simulink library "CAN_EV_lib"  (Simulink 7.5)
settings: Solver=ode45  StartTime=0.0  StopTime=10.0  RelTol=1e-3
values from neighbouring files (symbols this model uses):
  pOUTP_st_ChrgrPlugSwtACChrg_C = Simulink.Parameter    [CAN_par.m]
  pOUTP_st_ChrgrPlugSwtDCChrg_C = Simulink.Parameter    [CAN_par.m]
  pOUTP_st_ChrgrPlugSwtNoChrg_C = Simulink.Parameter    [CAN_par.m]
libraries: BaseOperationLib_Browser x6, simulink x1
settings Model: Creator=wuaibin  LastModifiedBy=wuaibin

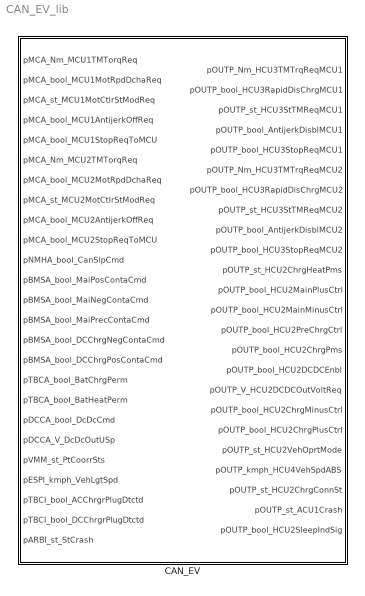
== system CAN_EV_lib ==
  CAN_EV : Subsystem

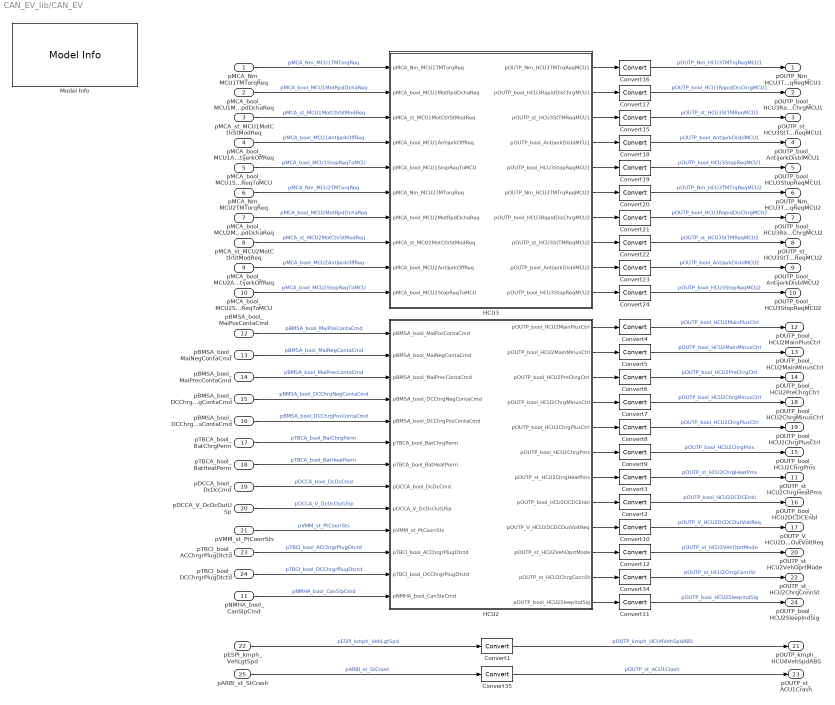
== system CAN_EV_lib/CAN_EV ==
  pMCA_Nm_MCU1TMTorqReq : Inport  OutDataType=fixdt(1, 16)  OutScaling=2^0
  pMCA_bool_MCU1MotRpdDchaReq : Inport  Port=2  OutDataType=fixdt(1, 16)  OutScaling=2^0
  pMCA_st_MCU1MotCtlrStModReq : Inport  Port=3  OutDataType=fixdt(1, 16)  OutScaling=2^0
  pMCA_bool_MCU1AntijerkOffReq : Inport  Port=4  OutDataType=fixdt(1, 16)  OutScaling=2^0
  pMCA_bool_MCU1StopReqToMCU : Inport  Port=5  OutDataType=fixdt(1, 16)  OutScaling=2^0
  pMCA_Nm_MCU2TMTorqReq : Inport  Port=6  OutDataType=fixdt(1, 16)  OutScaling=2^0
  pMCA_bool_MCU2MotRpdDchaReq : Inport  Port=7  OutDataType=fixdt(1, 16)  OutScaling=2^0
  pMCA_st_MCU2MotCtlrStModReq : Inport  Port=8  OutDataType=fixdt(1, 16)  OutScaling=2^0
  pMCA_bool_MCU2AntijerkOffReq : Inport  Port=9  OutDataType=fixdt(1, 16)  OutScaling=2^0
  pMCA_bool_MCU2StopReqToMCU : Inport  Port=10  OutDataType=fixdt(1, 16)  OutScaling=2^0
  pNMHA_bool_CanSlpCmd : Inport  Port=11  OutDataType=fixdt(1, 16)  OutScaling=2^0
  pBMSA_bool_MaiPosContaCmd : Inport  Port=12  OutDataType=fixdt(1, 16)  OutScaling=2^0
  pBMSA_bool_MaiNegContaCmd : Inport  Port=13  OutDataType=fixdt(1, 16)  OutScaling=2^0
  pBMSA_bool_MaiPrecContaCmd : Inport  Port=14  OutDataType=fixdt(1, 16)  OutScaling=2^0
  pBMSA_bool_DCChrgNegContaCmd : Inport  Port=15  OutDataType=fixdt(1, 16)  OutScaling=2^0
  pBMSA_bool_DCChrgPosContaCmd : Inport  Port=16  OutDataType=fixdt(1, 16)  OutScaling=2^0
  pTBCA_bool_BatChrgPerm : Inport  Port=17  OutDataType=fixdt(1, 16)  OutScaling=2^0
  pTBCA_bool_BatHeatPerm : Inport  Port=18  OutDataType=fixdt(1, 16)  OutScaling=2^0
  pDCCA_bool_DcDcCmd : Inport  Port=19  OutDataType=fixdt(1, 16)  OutScaling=2^0
  pDCCA_V_DcDcOutUSp : Inport  Port=20  OutDataType=fixdt(1, 16)  OutScaling=2^0
  pVMM_st_PtCoorrSts : Inport  Port=21  OutDataType=fixdt(1, 16)  OutScaling=2^0
  pESPI_kmph_VehLgtSpd : Inport  Port=22
  pTBCI_bool_ACChrgrPlugDtctd : Inport  Port=23  OutDataType=fixdt(1, 16)  OutScaling=2^0
  pTBCI_bool_DCChrgrPlugDtctd : Inport  Port=24  OutDataType=fixdt(1, 16)  OutScaling=2^0
  pARBI_st_StCrash : Inport  Port=25
  Convert{1..12,15..24,34..35} (24 alike) : DataTypeConversion  OutDataType=fixdt(1, 16)  OutScaling=2^0
  HCU2 : Subsystem
  HCU3 : Subsystem
  Model Info : simulink/Model-Wide Utilities/Model Info  SystemSampleTime=-1  InitialBlockCM=None  BlockCM=None  Frame=on  DisplayStringWithTags=Model Info\nCreated: %<Created>\nCreator: wuaibin  HorizontalTextAlignment=Center  LeftAlignmentValue=0.5  SourceBlockDiagram=HQEV_HCU  TagMaxNumber=20
  pOUTP_Nm_HCU3TMTrqReqMCU1 : Outport
  pOUTP_bool_HCU3RapidDisChrgMCU1 : Outport  Port=2
  pOUTP_st_HCU3StTMReqMCU1 : Outport  Port=3
  pOUTP_bool_AntijerkDisblMCU1 : Outport  Port=4
  pOUTP_bool_HCU3StopReqMCU1 : Outport  Port=5
  pOUTP_Nm_HCU3TMTrqReqMCU2 : Outport  Port=6
  pOUTP_bool_HCU3RapidDisChrgMCU2 : Outport  Port=7
  pOUTP_st_HCU3StTMReqMCU2 : Outport  Port=8
  pOUTP_bool_AntijerkDisblMCU2 : Outport  Port=9
  pOUTP_bool_HCU3StopReqMCU2 : Outport  Port=10
  pOUTP_st_HCU2ChrgHeatPms : Outport  Port=11  OutDataType=fixdt(1, 16)  OutScaling=2^0
  pOUTP_bool_HCU2MainPlusCtrl : Outport  Port=12  OutDataType=fixdt(1, 16)  OutScaling=2^0
  pOUTP_bool_HCU2MainMinusCtrl : Outport  Port=13  OutDataType=fixdt(1, 16)  OutScaling=2^0
  pOUTP_bool_HCU2PreChrgCtrl : Outport  Port=14  OutDataType=fixdt(1, 16)  OutScaling=2^0
  pOUTP_bool_HCU2ChrgPms : Outport  Port=15  OutDataType=fixdt(1, 16)  OutScaling=2^0
  pOUTP_bool_HCU2DCDCEnbl : Outport  Port=16  OutDataType=fixdt(1, 16)  OutScaling=2^0
  pOUTP_V_HCU2DCDCOutVoltReq : Outport  Port=17  OutDataType=fixdt(1, 16)  OutScaling=2^0
  pOUTP_bool_HCU2ChrgMinusCtrl : Outport  Port=18  OutDataType=fixdt(1, 16)  OutScaling=2^0
  pOUTP_bool_HCU2ChrgPlusCtrl : Outport  Port=19  OutDataType=fixdt(1, 16)  OutScaling=2^0
  pOUTP_st_HCU2VehOprtMode : Outport  Port=20  OutDataType=fixdt(1, 16)  OutScaling=2^0
  pOUTP_kmph_HCU4VehSpdABS : Outport  Port=21
  pOUTP_st_HCU2ChrgConnSt : Outport  Port=22  OutDataType=fixdt(1, 16)  OutScaling=2^0
  pOUTP_st_ACU1Crash : Outport  Port=23
  pOUTP_bool_HCU2SleepIndSig : Outport  Port=24  OutDataType=fixdt(1, 16)  OutScaling=2^0
  wires:
  Convert11/1 -> pOUTP_bool_HCU2SleepIndSig/1  "pOUTP_bool_HCU2SleepIndSig"
  HCU2/12(pOUTP_bool_HCU2SleepIndSig) -> Convert11/1
  pNMHA_bool_CanSlpCmd/1 -> HCU2/13(pNMHA_bool_CanSlpCmd)  "pNMHA_bool_CanSlpCmd"
  pARBI_st_StCrash/1 -> Convert35/1  "pARBI_st_StCrash"
  Convert35/1 -> pOUTP_st_ACU1Crash/1  "pOUTP_st_ACU1Crash"
  Convert24/1 -> pOUTP_bool_HCU3StopReqMCU2/1  "pOUTP_bool_HCU3StopReqMCU2"
  Convert23/1 -> pOUTP_bool_AntijerkDisblMCU2/1  "pOUTP_bool_AntijerkDisblMCU2"
  Convert22/1 -> pOUTP_st_HCU3StTMReqMCU2/1  "pOUTP_st_HCU3StTMReqMCU2"
  Convert21/1 -> pOUTP_bool_HCU3RapidDisChrgMCU2/1  "pOUTP_bool_HCU3RapidDisChrgMCU2"
  Convert20/1 -> pOUTP_Nm_HCU3TMTrqReqMCU2/1  "pOUTP_Nm_HCU3TMTrqReqMCU2"
  Convert19/1 -> pOUTP_bool_HCU3StopReqMCU1/1  "pOUTP_bool_HCU3StopReqMCU1"
  Convert18/1 -> pOUTP_bool_AntijerkDisblMCU1/1  "pOUTP_bool_AntijerkDisblMCU1"
  Convert15/1 -> pOUTP_st_HCU3StTMReqMCU1/1  "pOUTP_st_HCU3StTMReqMCU1"
  Convert17/1 -> pOUTP_bool_HCU3RapidDisChrgMCU1/1  "pOUTP_bool_HCU3RapidDisChrgMCU1"
  Convert16/1 -> pOUTP_Nm_HCU3TMTrqReqMCU1/1  "pOUTP_Nm_HCU3TMTrqReqMCU1"
  Convert12/1 -> pOUTP_st_HCU2VehOprtMode/1  "pOUTP_st_HCU2VehOprtMode"
  Convert10/1 -> pOUTP_V_HCU2DCDCOutVoltReq/1  "pOUTP_V_HCU2DCDCOutVoltReq"
  Convert9/1 -> pOUTP_bool_HCU2ChrgPms/1  "pOUTP_bool_HCU2ChrgPms"
  Convert8/1 -> pOUTP_bool_HCU2ChrgPlusCtrl/1  "pOUTP_bool_HCU2ChrgPlusCtrl"
  Convert7/1 -> pOUTP_bool_HCU2ChrgMinusCtrl/1  "pOUTP_bool_HCU2ChrgMinusCtrl"
  Convert6/1 -> pOUTP_bool_HCU2PreChrgCtrl/1  "pOUTP_bool_HCU2PreChrgCtrl"
  Convert5/1 -> pOUTP_bool_HCU2MainMinusCtrl/1  "pOUTP_bool_HCU2MainMinusCtrl"
  Convert4/1 -> pOUTP_bool_HCU2MainPlusCtrl/1  "pOUTP_bool_HCU2MainPlusCtrl"
  Convert3/1 -> pOUTP_st_HCU2ChrgHeatPms/1  "pOUTP_st_HCU2ChrgHeatPms"
  Convert2/1 -> pOUTP_bool_HCU2DCDCEnbl/1  "pOUTP_bool_HCU2DCDCEnbl"
  pTBCI_bool_DCChrgrPlugDtctd/1 -> HCU2/12(pTBCI_bool_DCChrgrPlugDtctd)  "pTBCI_bool_DCChrgrPlugDtctd"
  pTBCI_bool_ACChrgrPlugDtctd/1 -> HCU2/11(pTBCI_bool_ACChrgrPlugDtctd)  "pTBCI_bool_ACChrgrPlugDtctd"
  Convert34/1 -> pOUTP_st_HCU2ChrgConnSt/1  "pOUTP_st_HCU2ChrgConnSt"
  HCU2/11(pOUTP_st_HCU2ChrgConnSt) -> Convert34/1
  Convert1/1 -> pOUTP_kmph_HCU4VehSpdABS/1  "pOUTP_kmph_HCU4VehSpdABS"
  pESPI_kmph_VehLgtSpd/1 -> Convert1/1  "pESPI_kmph_VehLgtSpd"
  HCU2/10(pOUTP_st_HCU2VehOprtMode) -> Convert12/1
  pVMM_st_PtCoorrSts/1 -> HCU2/10(pVMM_st_PtCoorrSts)  "pVMM_st_PtCoorrSts"
  HCU3/7(pOUTP_bool_HCU3RapidDisChrgMCU2) -> Convert21/1
  HCU3/8(pOUTP_st_HCU3StTMReqMCU2) -> Convert22/1
  HCU3/9(pOUTP_bool_AntijerkDisblMCU2) -> Convert23/1
  HCU3/10(pOUTP_bool_HCU3StopReqMCU2) -> Convert24/1
  HCU3/1(pOUTP_Nm_HCU3TMTrqReqMCU1) -> Convert16/1
  HCU3/2(pOUTP_bool_HCU3RapidDisChrgMCU1) -> Convert17/1
  HCU3/3(pOUTP_st_HCU3StTMReqMCU1) -> Convert15/1
  HCU3/4(pOUTP_bool_AntijerkDisblMCU1) -> Convert18/1
  HCU3/5(pOUTP_bool_HCU3StopReqMCU1) -> Convert19/1
  HCU3/6(pOUTP_Nm_HCU3TMTrqReqMCU2) -> Convert20/1
  pMCA_bool_MCU2StopReqToMCU/1 -> HCU3/10(pMCA_bool_MCU2StopReqToMCU)  "pMCA_bool_MCU2StopReqToMCU"
  pMCA_bool_MCU2AntijerkOffReq/1 -> HCU3/9(pMCA_bool_MCU2AntijerkOffReq)  "pMCA_bool_MCU2AntijerkOffReq"
  pMCA_st_MCU2MotCtlrStModReq/1 -> HCU3/8(pMCA_st_MCU2MotCtlrStModReq)  "pMCA_st_MCU2MotCtlrStModReq"
  pMCA_bool_MCU2MotRpdDchaReq/1 -> HCU3/7(pMCA_bool_MCU2MotRpdDchaReq)  "pMCA_bool_MCU2MotRpdDchaReq"
  pMCA_Nm_MCU1TMTorqReq/1 -> HCU3/1(pMCA_Nm_MCU1TMTorqReq)  "pMCA_Nm_MCU1TMTorqReq"
  pMCA_bool_MCU1MotRpdDchaReq/1 -> HCU3/2(pMCA_bool_MCU1MotRpdDchaReq)  "pMCA_bool_MCU1MotRpdDchaReq"
  pMCA_st_MCU1MotCtlrStModReq/1 -> HCU3/3(pMCA_st_MCU1MotCtlrStModReq)  "pMCA_st_MCU1MotCtlrStModReq"
  pMCA_bool_MCU1AntijerkOffReq/1 -> HCU3/4(pMCA_bool_MCU1AntijerkOffReq)  "pMCA_bool_MCU1AntijerkOffReq"
  pMCA_bool_MCU1StopReqToMCU/1 -> HCU3/5(pMCA_bool_MCU1StopReqToMCU)  "pMCA_bool_MCU1StopReqToMCU"
  pMCA_Nm_MCU2TMTorqReq/1 -> HCU3/6(pMCA_Nm_MCU2TMTorqReq)  "pMCA_Nm_MCU2TMTorqReq"
  pBMSA_bool_MaiPosContaCmd/1 -> HCU2/1(pBMSA_bool_MaiPosContaCmd)  "pBMSA_bool_MaiPosContaCmd"
  pBMSA_bool_MaiNegContaCmd/1 -> HCU2/2(pBMSA_bool_MaiNegContaCmd)  "pBMSA_bool_MaiNegContaCmd"
  pBMSA_bool_MaiPrecContaCmd/1 -> HCU2/3(pBMSA_bool_MaiPrecContaCmd)  "pBMSA_bool_MaiPrecContaCmd"
  pTBCA_bool_BatChrgPerm/1 -> HCU2/6(pTBCA_bool_BatChrgPerm)  "pTBCA_bool_BatChrgPerm"
  pTBCA_bool_BatHeatPerm/1 -> HCU2/7(pTBCA_bool_BatHeatPerm)  "pTBCA_bool_BatHeatPerm"
  HCU2/7(pOUTP_st_HCU2ChrgHeatPms) -> Convert3/1
  HCU2/1(pOUTP_bool_HCU2MainPlusCtrl) -> Convert4/1
  HCU2/2(pOUTP_bool_HCU2MainMinusCtrl) -> Convert5/1
  HCU2/3(pOUTP_bool_HCU2PreChrgCtrl) -> Convert6/1
  HCU2/6(pOUTP_bool_HCU2ChrgPms) -> Convert9/1
  HCU2/8(pOUTP_bool_HCU2DCDCEnbl) -> Convert2/1
  HCU2/9(pOUTP_V_HCU2DCDCOutVoltReq) -> Convert10/1
  pDCCA_bool_DcDcCmd/1 -> HCU2/8(pDCCA_bool_DcDcCmd)  "pDCCA_bool_DcDcCmd"
  pDCCA_V_DcDcOutUSp/1 -> HCU2/9(pDCCA_V_DcDcOutUSp)  "pDCCA_V_DcDcOutUSp"
  pBMSA_bool_DCChrgNegContaCmd/1 -> HCU2/4(pBMSA_bool_DCChrgNegContaCmd)  "pBMSA_bool_DCChrgNegContaCmd"
  pBMSA_bool_DCChrgPosContaCmd/1 -> HCU2/5(pBMSA_bool_DCChrgPosContaCmd)  "pBMSA_bool_DCChrgPosContaCmd"
  HCU2/4(pOUTP_bool_HCU2ChrgMinusCtrl) -> Convert7/1
  HCU2/5(pOUTP_bool_HCU2ChrgPlusCtrl) -> Convert8/1

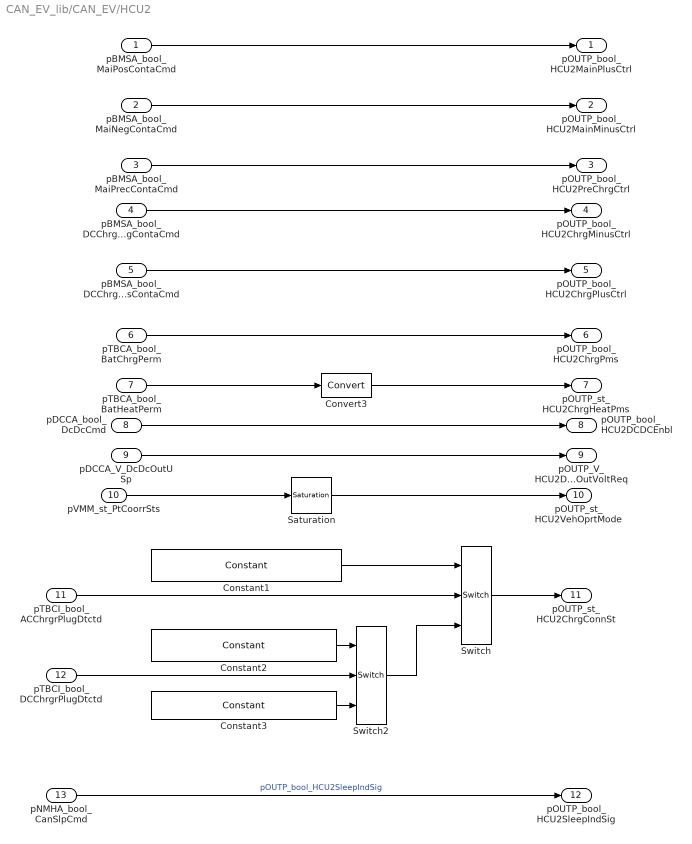
== system CAN_EV_lib/CAN_EV/HCU2 ==
  pBMSA_bool_MaiPosContaCmd : Inport  OutDataType=fixdt(1, 16)  OutScaling=2^0
  pBMSA_bool_MaiNegContaCmd : Inport  Port=2  OutDataType=fixdt(1, 16)  OutScaling=2^0
  pBMSA_bool_MaiPrecContaCmd : Inport  Port=3  OutDataType=fixdt(1, 16)  OutScaling=2^0
  pBMSA_bool_DCChrgNegContaCmd : Inport  Port=4  OutDataType=fixdt(1, 16)  OutScaling=2^0
  pBMSA_bool_DCChrgPosContaCmd : Inport  Port=5  OutDataType=fixdt(1, 16)  OutScaling=2^0
  pTBCA_bool_BatChrgPerm : Inport  Port=6  OutDataType=fixdt(1, 16)  OutScaling=2^0
  pTBCA_bool_BatHeatPerm : Inport  Port=7  OutDataType=fixdt(1, 16)  OutScaling=2^0
  pDCCA_bool_DcDcCmd : Inport  Port=8  OutDataType=fixdt(1, 16)  OutScaling=2^0
  pDCCA_V_DcDcOutUSp : Inport  Port=9  OutDataType=fixdt(1, 16)  OutScaling=2^0
  pVMM_st_PtCoorrSts : Inport  Port=10
  pTBCI_bool_ACChrgrPlugDtctd : Inport  Port=11  OutDataType=fixdt(1, 16)  OutScaling=2^0
  pTBCI_bool_DCChrgrPlugDtctd : Inport  Port=12  OutDataType=fixdt(1, 16)  OutScaling=2^0
  pNMHA_bool_CanSlpCmd : Inport  Port=13  OutDataType=fixdt(1, 16)  OutScaling=2^0
  Constant1 : BaseOperationLib_Browser/Sources&Sinks/Constant  Value=pOUTP_st_ChrgrPlugSwtACChrg_C  OutMin=[]  OutMax=[]  OutDataType=fixdt(1, 16)  ConRadixGroup=Use specified scaling  OutScaling=2^0  OutDataTypeStr=Inherit: Inherit from 'Constant value'
  Constant2 : BaseOperationLib_Browser/Sources&Sinks/Constant  Value=pOUTP_st_ChrgrPlugSwtDCChrg_C  OutMin=[]  OutMax=[]  OutDataType=fixdt(1, 16)  ConRadixGroup=Use specified scaling  OutScaling=2^0  OutDataTypeStr=Inherit: Inherit from 'Constant value'
  Constant3 : BaseOperationLib_Browser/Sources&Sinks/Constant  Value=pOUTP_st_ChrgrPlugSwtNoChrg_C  OutMin=[]  OutMax=[]  OutDataType=fixdt(1, 16)  ConRadixGroup=Use specified scaling  OutScaling=2^0  OutDataTypeStr=Inherit: Inherit from 'Constant value'
  Convert3 : DataTypeConversion  OutDataType=fixdt(1, 16)  OutScaling=2^0
  Saturation : BaseOperationLib_Browser/Discontinuities Unchanged/Saturation  UpperLimit=15  LowerLimit=0  OutMin=[]  OutMax=[]  OutDataType=fixdt(1, 16)  OutScaling=2^0
      settings: AttributesFormatString=ULim:%<UpperLimit>\nLLim:%<LowerLimit>
  Switch : BaseOperationLib_Browser/Signal Routing Changed/Switch  Criteria=u2 ~= 0  Threshold=1  InputSameDT=on  OutMin=[]  OutMax=[]  OutDataType=fixdt(1,16,0)  OutScaling=[]  SaturateOnIntegerOverflow=on
  Switch2 : BaseOperationLib_Browser/Signal Routing Changed/Switch  Criteria=u2 ~= 0  Threshold=1  InputSameDT=on  OutMin=[]  OutMax=[]  OutDataType=fixdt(1,16,0)  OutScaling=[]  SaturateOnIntegerOverflow=on
  pOUTP_bool_HCU2MainPlusCtrl : Outport  OutDataType=fixdt(1, 16)  OutScaling=2^0
  pOUTP_bool_HCU2MainMinusCtrl : Outport  Port=2  OutDataType=fixdt(1, 16)  OutScaling=2^0
  pOUTP_bool_HCU2PreChrgCtrl : Outport  Port=3  OutDataType=fixdt(1, 16)  OutScaling=2^0
  pOUTP_bool_HCU2ChrgMinusCtrl : Outport  Port=4  OutDataType=fixdt(1, 16)  OutScaling=2^0
  pOUTP_bool_HCU2ChrgPlusCtrl : Outport  Port=5  OutDataType=fixdt(1, 16)  OutScaling=2^0
  pOUTP_bool_HCU2ChrgPms : Outport  Port=6  OutDataType=fixdt(1, 16)  OutScaling=2^0
  pOUTP_st_HCU2ChrgHeatPms : Outport  Port=7  OutDataType=fixdt(1, 16)  OutScaling=2^0
  pOUTP_bool_HCU2DCDCEnbl : Outport  Port=8  OutDataType=fixdt(1, 16)  OutScaling=2^0
  pOUTP_V_HCU2DCDCOutVoltReq : Outport  Port=9  OutDataType=fixdt(1, 16)  OutScaling=2^0
  pOUTP_st_HCU2VehOprtMode : Outport  Port=10
  pOUTP_st_HCU2ChrgConnSt : Outport  Port=11  OutDataType=fixdt(1, 16)  OutScaling=2^0
  pOUTP_bool_HCU2SleepIndSig : Outport  Port=12  OutDataType=fixdt(1, 16)  OutScaling=2^0
  wires:
  pNMHA_bool_CanSlpCmd/1 -> pOUTP_bool_HCU2SleepIndSig/1  "pOUTP_bool_HCU2SleepIndSig"
  Convert3/1 -> pOUTP_st_HCU2ChrgHeatPms/1
  pTBCI_bool_ACChrgrPlugDtctd/1 -> Switch/2
  Switch/1 -> pOUTP_st_HCU2ChrgConnSt/1
  Constant1/1 -> Switch/1
  Switch2/1 -> Switch/3
  Constant2/1 -> Switch2/1
  pTBCI_bool_DCChrgrPlugDtctd/1 -> Switch2/2
  Constant3/1 -> Switch2/3
  pVMM_st_PtCoorrSts/1 -> Saturation/1
  pBMSA_bool_MaiPosContaCmd/1 -> pOUTP_bool_HCU2MainPlusCtrl/1
  pBMSA_bool_MaiNegContaCmd/1 -> pOUTP_bool_HCU2MainMinusCtrl/1
  pBMSA_bool_MaiPrecContaCmd/1 -> pOUTP_bool_HCU2PreChrgCtrl/1
  pTBCA_bool_BatChrgPerm/1 -> pOUTP_bool_HCU2ChrgPms/1
  pTBCA_bool_BatHeatPerm/1 -> Convert3/1
  pDCCA_V_DcDcOutUSp/1 -> pOUTP_V_HCU2DCDCOutVoltReq/1
  pDCCA_bool_DcDcCmd/1 -> pOUTP_bool_HCU2DCDCEnbl/1
  pBMSA_bool_DCChrgNegContaCmd/1 -> pOUTP_bool_HCU2ChrgMinusCtrl/1
  pBMSA_bool_DCChrgPosContaCmd/1 -> pOUTP_bool_HCU2ChrgPlusCtrl/1
  Saturation/1 -> pOUTP_st_HCU2VehOprtMode/1

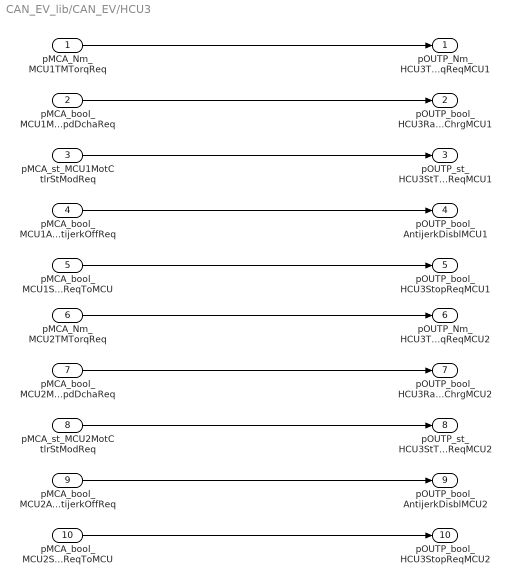
== system CAN_EV_lib/CAN_EV/HCU3 ==
  pMCA_Nm_MCU1TMTorqReq : Inport  OutDataType=fixdt(1, 16)  OutScaling=2^0
  pMCA_bool_MCU1MotRpdDchaReq : Inport  Port=2  OutDataType=fixdt(1, 16)  OutScaling=2^0
  pMCA_st_MCU1MotCtlrStModReq : Inport  Port=3  OutDataType=fixdt(1, 16)  OutScaling=2^0
  pMCA_bool_MCU1AntijerkOffReq : Inport  Port=4  OutDataType=fixdt(1, 16)  OutScaling=2^0
  pMCA_bool_MCU1StopReqToMCU : Inport  Port=5  OutDataType=fixdt(1, 16)  OutScaling=2^0
  pMCA_Nm_MCU2TMTorqReq : Inport  Port=6  OutDataType=fixdt(1, 16)  OutScaling=2^0
  pMCA_bool_MCU2MotRpdDchaReq : Inport  Port=7  OutDataType=fixdt(1, 16)  OutScaling=2^0
  pMCA_st_MCU2MotCtlrStModReq : Inport  Port=8  OutDataType=fixdt(1, 16)  OutScaling=2^0
  pMCA_bool_MCU2AntijerkOffReq : Inport  Port=9  OutDataType=fixdt(1, 16)  OutScaling=2^0
  pMCA_bool_MCU2StopReqToMCU : Inport  Port=10  OutDataType=fixdt(1, 16)  OutScaling=2^0
  pOUTP_Nm_HCU3TMTrqReqMCU1 : Outport
  pOUTP_bool_HCU3RapidDisChrgMCU1 : Outport  Port=2
  pOUTP_st_HCU3StTMReqMCU1 : Outport  Port=3
  pOUTP_bool_AntijerkDisblMCU1 : Outport  Port=4
  pOUTP_bool_HCU3StopReqMCU1 : Outport  Port=5
  pOUTP_Nm_HCU3TMTrqReqMCU2 : Outport  Port=6
  pOUTP_bool_HCU3RapidDisChrgMCU2 : Outport  Port=7
  pOUTP_st_HCU3StTMReqMCU2 : Outport  Port=8
  pOUTP_bool_AntijerkDisblMCU2 : Outport  Port=9
  pOUTP_bool_HCU3StopReqMCU2 : Outport  Port=10
  wires:
  pMCA_Nm_MCU1TMTorqReq/1 -> pOUTP_Nm_HCU3TMTrqReqMCU1/1
  pMCA_bool_MCU1MotRpdDchaReq/1 -> pOUTP_bool_HCU3RapidDisChrgMCU1/1
  pMCA_st_MCU1MotCtlrStModReq/1 -> pOUTP_st_HCU3StTMReqMCU1/1
  pMCA_bool_MCU1AntijerkOffReq/1 -> pOUTP_bool_AntijerkDisblMCU1/1
  pMCA_bool_MCU1StopReqToMCU/1 -> pOUTP_bool_HCU3StopReqMCU1/1
  pMCA_Nm_MCU2TMTorqReq/1 -> pOUTP_Nm_HCU3TMTrqReqMCU2/1
  pMCA_bool_MCU2MotRpdDchaReq/1 -> pOUTP_bool_HCU3RapidDisChrgMCU2/1
  pMCA_st_MCU2MotCtlrStModReq/1 -> pOUTP_st_HCU3StTMReqMCU2/1
  pMCA_bool_MCU2AntijerkOffReq/1 -> pOUTP_bool_AntijerkDisblMCU2/1
  pMCA_bool_MCU2StopReqToMCU/1 -> pOUTP_bool_HCU3StopReqMCU2/1
